simulink model "Proj2"  (R2025a)
settings: Solver=FixedStepDiscrete  StartTime=0.0  StopTime=100.0  FixedStep=0.01  RelTol=1e-3  EnableMultiTasking=on
undefined symbols (not defined in the file): A_total, b, c, DiscIntNeverNeededParam, T_dif, T_get, T_off, T_on, x0
settings Model: SILPILModeSetting=veronly  CodeVerificationMode=processor-in-the-loop (pil)  ExtModeTrigDuration=2  Creator=Lenovo  LastModifiedBy=Sina
settings SolverCC: AutoInsertRateTranBlk=on
settings OptimizationCC: EnhancedBackFolding=on  PassReuseOutputArgsAs=Individual arguments  ZeroExternalMemoryAtStartup=off  ZeroInternalMemoryAtStartup=off  MaxStackSize=64  OptimizeBlockOrder=speed  DifferentSizesBufferReuse=on  OptimizationCustomize=off  EfficientTunableParamExpr=on
settings DebuggingCC: ParameterTunabilityLossMsg=error
settings HardwareCC: ProdBitPerInt=16.0  ProdBitPerPointer=16.0  ProdBitPerSizeT=16.0  ProdBitPerPtrDiffT=16.0  ProdLargestAtomicFloat=None  ProdWordSize=8.0  ProdHWDeviceType=Atmel->AVR
settings SFSimCC: MATLABDynamicMemAlloc=off
settings RTWCC: SystemTargetFile=ert.tlc  HardwareBoard=Arduino Uno  GenCodeOnly=on  TemplateMakefile=ert_default_tmf  Toolchain=Arduino AVR  BuildConfiguration=Faster Runs  Description=Embedded Coder
settings CodeAppCC: ForceParamTrailComments=on  IgnoreCustomStorageClasses=off  OperatorAnnotations=on  SimulinkDataObjDesc=on  SFDataObjDesc=on  InsertBlockDesc=on
settings ERTTargetCC: ExtModeTransport=3.0  ExtModeAutomaticAllocSize=off  ExtModeStaticAllocSize=250.0  InlinedParameterPlacement=Hierarchical  SupportContinuousTime=on  SupportVariableSizeSignals=on
settings ConfigComp: CovEnable=on  RecordCoverage=on  CovModelRefEnable=on

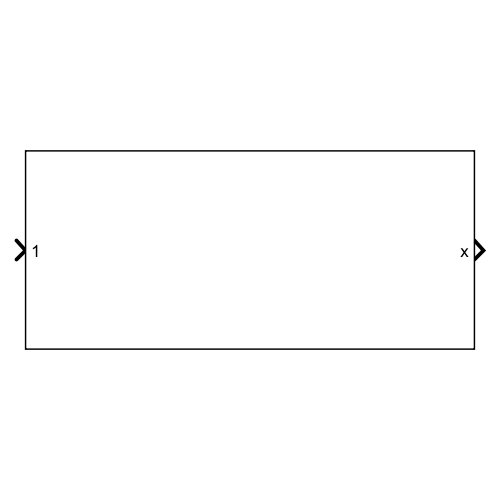
[thumbnail: Simulink's stored preview of the top-level diagram]
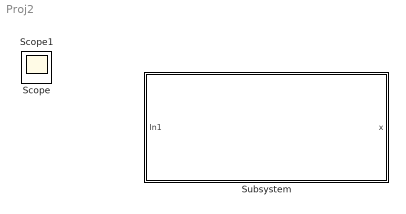
== system Proj2 ==
  Subsystem : Subsystem
  Scope : Scope
      settings: ActiveDisplayYMinimum=12.503923149289818  ActiveDisplayYMaximum=22.756897729507291
  Scope1 : Scope
      settings: ActiveDisplayYMinimum=-4.0864043294794055  ActiveDisplayYMaximum=5.4144619829626475

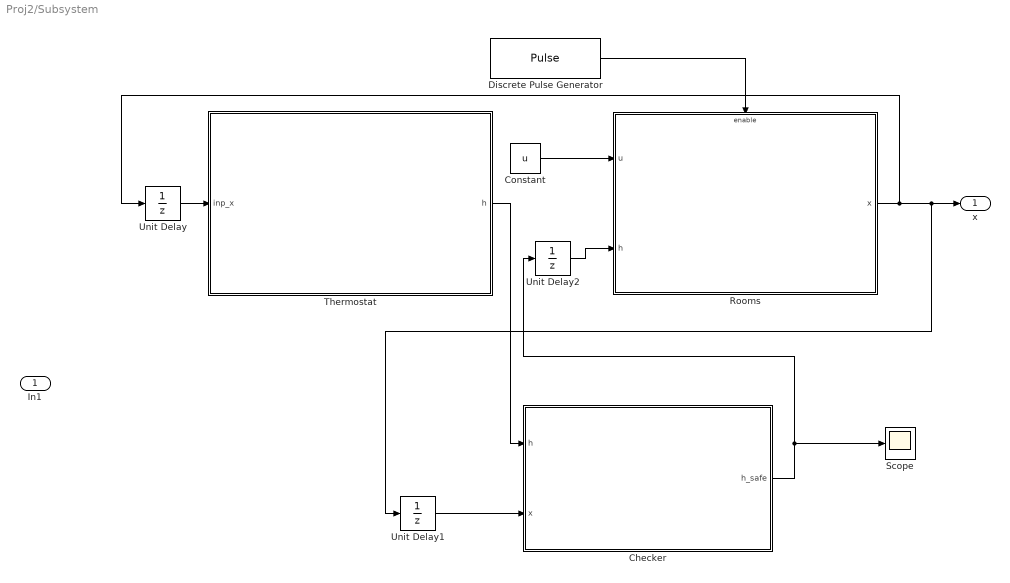
== system Proj2/Subsystem ==
  In1 : Inport
  Checker : Subsystem
  Constant : Constant  Value=u
  Discrete Pulse Generator : DiscretePulseGenerator  PulseType=Time based  Period=1  PulseWidth=50
  Rooms : Subsystem
  Scope : Scope
      settings: ActiveDisplayYMinimum=-0.12499999999999997  ActiveDisplayYMaximum=1.125  DataLoggingVariableName=ScopeData2
  Thermostat : Subsystem
  Unit Delay : UnitDelay  SampleTime=-1  HasFrameUpgradeWarning=on
  Unit Delay1 : UnitDelay  SampleTime=-1  HasFrameUpgradeWarning=on
  Unit Delay2 : UnitDelay  SampleTime=-1  HasFrameUpgradeWarning=on
  x : Outport
  wires:
  Constant/1 -> Rooms/1(u)
  Rooms/1(x) -> Unit Delay/1, Unit Delay1/1, x/1
  Discrete Pulse Generator/1 -> Rooms/Enable
  Unit Delay/1 -> Thermostat/1(inp_x)
  Unit Delay2/1 -> Rooms/2(h)
  Checker/1(h_safe) -> Scope/1, Unit Delay2/1
  Thermostat/1(h) -> Checker/1(h)
  Unit Delay1/1 -> Checker/2(x)

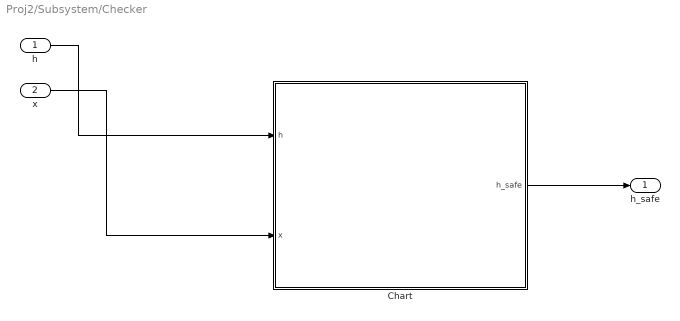
== system Proj2/Subsystem/Checker ==
  h : Inport
  x : Inport  Port=2
  Chart : Stateflow chart  TreatAsAtomicUnit=on
  h_safe : Outport
  wires:
  h/1 -> Chart/1(h)
  Chart/1(h_safe) -> h_safe/1
  x/1 -> Chart/2(x)

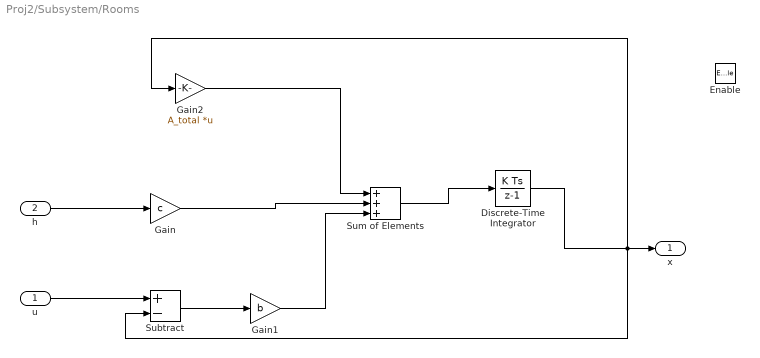
== system Proj2/Subsystem/Rooms ==
  u : Inport
  h : Inport  Port=2
  Enable : EnablePort
  Discrete-Time Integrator : DiscreteIntegrator  InitialCondition=x0  SampleTime=-1  ICPrevOutput=DiscIntNeverNeededParam  ICPrevScaledInput=DiscIntNeverNeededParam
  Gain : Gain  Gain=c
  Gain1 : Gain  Gain=b
  Gain2 : Gain  Gain=A_total  Multiplication=Matrix(K*u)
  Subtract : Sum  Inputs=+-
  Sum of Elements : Sum  Inputs=+++
  x : Outport
  wires:
  Discrete-Time Integrator/1 -> Gain2/1, Subtract/2, x/1
  h/1 -> Gain/1
  u/1 -> Subtract/1
  Subtract/1 -> Gain1/1
  Gain2/1 -> Sum of Elements/1
  Gain/1 -> Sum of Elements/2
  Gain1/1 -> Sum of Elements/3
  Sum of Elements/1 -> Discrete-Time Integrator/1

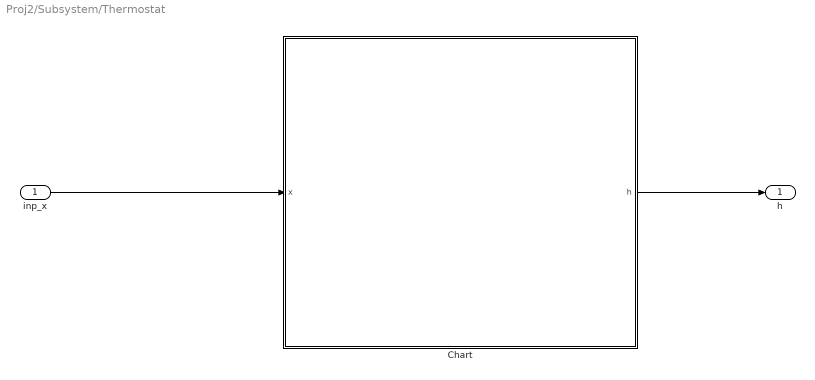
== system Proj2/Subsystem/Thermostat ==
  inp_x : Inport
  Chart : Stateflow chart  TreatAsAtomicUnit=on
  h : Outport
  wires:
  Chart/1(h) -> h/1
  inp_x/1 -> Chart/1(x)

== stateflow chart Proj2/Subsystem/Checker/Chart ==
  state Block
  state Safe
  Block -> Safe [order 1] : [sum(h)<=2]{h_safe = h}
  Safe -> Safe [order 2] : [sum(h)<=2]{h_safe = h}
  (default) -> Block
  Block -> Block [order 2] : [sum(h) > 2 || any((h==1 & x>=T_off) | (h==0 & x<=T_on))]
  Safe -> Block [order 1] : [sum(h) > 2 || any((h==1 & x>=T_off) | (h==0 & x<=T_on))]
  data: h input; h_safe output size=[4 1] =[0;0;0;0]; T_off parameter; T_on parameter; x input

== stateflow chart Proj2/Subsystem/Thermostat/Chart ==
  settings: updateMethod=DISCRETE  sampleTime=0.01
  state S0110
    state S3
    (default) -> S0110.S3
    S0110.S3 -> S0110.S3 [order 4] : [x(2)>=T_off(2) && h(2) == 1]{h(2) = 0;}
    S0110.S3 -> S0110.S3 [order 3] : [x(2) <=T_on(2) && h(2) == 0]{h(2) = 1;}
    S0110.S3 -> S0110.S3 [order 2] : [x(3) <=T_on(3) && h(3) == 0]{h(3) = 1;}
    S0110.S3 -> S0110.S3 [order 1] : [x(3)>=T_off(3) && h(3) == 1]{h(3) = 0;}
  state S1100
    state S3
    (default) -> S1100.S3
    S1100.S3 -> S1100.S3 [order 4] : [x(2)>=T_off(2) && h(2) == 1]{h(2) = 0;}
    S1100.S3 -> S1100.S3 [order 3] : [x(2) <=T_on(2) && h(2) == 0]{h(2) = 1;}
    S1100.S3 -> S1100.S3 [order 2] : [x(1) <=T_on(1) && h(1) == 0]{h(1) = 1;}
    S1100.S3 -> S1100.S3 [order 1] : [x(1)>=T_off(1) && h(1) == 1]{h(1) = 0;}
  state S0011
    state S3
    (default) -> S0011.S3
    S0011.S3 -> S0011.S3 [order 4] : [x(4)>=T_off(4) && h(4) == 1]{h(4) = 0;}
    S0011.S3 -> S0011.S3 [order 3] : [x(4) <=T_on(4) && h(4) == 0]{h(4) = 1;}
    S0011.S3 -> S0011.S3 [order 2] : [x(3) <=T_on(3) && h(3) == 0]{h(3) = 1;}
    S0011.S3 -> S0011.S3 [order 1] : [x(3)>=T_off(3) && h(3) == 1]{h(3) = 0;}
  state S0101
    state S3
    (default) -> S0101.S3
    S0101.S3 -> S0101.S3 [order 4] : [x(2)>=T_off(2) && h(2) == 1]{h(2) = 0;}
    S0101.S3 -> S0101.S3 [order 3] : [x(2) <=T_on(2) && h(2) == 0]{h(2) = 1;}
    S0101.S3 -> S0101.S3 [order 2] : [x(4) <=T_on(4) && h(4) == 0]{h(4) = 1;}
    S0101.S3 -> S0101.S3 [order 1] : [x(4)>=T_off(4) && h(4) == 1]{h(4) = 0;}
  state S1010
    state S3
    (default) -> S1010.S3
    S1010.S3 -> S1010.S3 [order 4] : [x(3)>=T_off(3) && h(3) == 1]{h(3) = 0;}
    S1010.S3 -> S1010.S3 [order 3] : [x(3) <=T_on(3) && h(3) == 0]{h(3) = 1;}
    S1010.S3 -> S1010.S3 [order 2] : [x(1) <=T_on(1) && h(1) == 0]{h(1) = 1;}
    S1010.S3 -> S1010.S3 [order 1] : [x(1)>=T_off(1) && h(1) == 1]{h(1) = 0;}
  state S1001
    state S3
    (default) -> S1001.S3
    S1001.S3 -> S1001.S3 [order 2] : [x(4)>=T_off(4) && h(4) == 1]{h(4) = 0;}
    S1001.S3 -> S1001.S3 [order 1] : [x(4) <=T_on(4) && h(4) == 0]{h(4) = 1;}
    S1001.S3 -> S1001.S3 [order 4] : [x(1) <=T_on(1) && h(1) == 0]{h(1) = 1;}
    S1001.S3 -> S1001.S3 [order 3] : [x(1)>=T_off(1) && h(1) == 1]{h(1) = 0;}
  S0101 -> S0110 [order 1] : [x(3) <=T_get(3) && x(4) - x(3) >= T_dif(3)]{h(4) = 0; h(3) = 1;}
  (default) -> S0110
  S0110 -> S0101 [order 2] : [x(4) <=T_get(4) && x(3) - x(4) >= T_dif(4)]{h(3) = 0; h(4) = 1;}
  S0110 -> S1010 [order 3] : [x(1) <=T_get(1) && x(2) - x(1) >= T_dif(1)]{h(2) = 0; h(1) = 1;}
  S0110 -> S1100 [order 1] : [x(1) <=T_get(1) && x(3) - x(1) >= T_dif(1)]{h(3) = 0; h(1) = 1;}
  S1100 -> S0110 [order 1] : [x(3) <=T_get(3) && x(1) - x(3) >= T_dif(3)]{h(1) = 0; h(3) = 1;}
  S1010 -> S0110 [order 1] : [x(2) <=T_get(2) && x(1) - x(2) >= T_dif(2)]{h(1) = 0; h(2) = 1;}
  S0110 -> S0011 [order 4] : [x(4) <=T_get(4) && x(2) - x(4) >= T_dif(4)]{h(2) = 0; h(4) = 1;}
  S0011 -> S0110 [order 1] : [x(2) <=T_get(2) && x(4) - x(2) >= T_dif(2)]{h(4) = 0; h(2) = 1;}
  S1001 -> S0011 [order 4] : [x(3) <=T_get(3) && x(1) - x(3) >= T_dif(3)]{h(1) = 0; h(3) = 1;}
  S0011 -> S0101 [order 3] : [x(2) <=T_get(2) && x(3) - x(2) >= T_dif(2)]{h(3) = 0; h(2) = 1;}
  S1010 -> S1100 [order 4] : [x(2) <=T_get(2) && x(3) - x(2) >= T_dif(2)]{h(3) = 0; h(2) = 1;}
  S0101 -> S1100 [order 2] : [x(1) <=T_get(1) && x(4) - x(1) >= T_dif(1)]{h(4) = 0; h(1) = 1;}
  S1001 -> S1100 [order 3] : [x(2) <=T_get(2) && x(4) - x(2) >= T_dif(2)]{h(4) = 0; h(2) = 1;}
  S1100 -> S1001 [order 4] : [x(4) <=T_get(4) && x(2) - x(4) >= T_dif(4)]{h(2) = 0; h(4) = 1;}
  S1100 -> S0101 [order 2] : [x(4) <=T_get(4) && x(1) - x(4) >= T_dif(4)]{h(1) = 0; h(4) = 1;}
  S1100 -> S1010 [order 3] : [x(3) <=T_get(3) && x(2) - x(3) >= T_dif(3)]{h(2) = 0; h(3) = 1;}
  S0101 -> S0011 [order 4] : [x(3) <=T_get(3) && x(2) - x(3) >= T_dif(3)]{h(2) = 0; h(3) = 1;}
  S0011 -> S1001 [order 4] : [x(1) <=T_get(1) && x(3) - x(1) >= T_dif(1)]{h(3) = 0; h(1) = 1;}
  S1010 -> S0011 [order 2] : [x(4) <=T_get(4) && x(1) - x(4) >= T_dif(4)]{h(1) = 0; h(4) = 1;}
  S0011 -> S1010 [order 2] : [x(1) <=T_get(1) && x(4) - x(1) >= T_dif(1)]{h(4) = 0; h(1) = 1;}
  S1001 -> S0101 [order 1] : [x(2) <=T_get(2) && x(1) - x(2) >= T_dif(2)]{h(1) = 0; h(2) = 1;}
  S1001 -> S1010 [order 2] : [x(3) <=T_get(3) && x(4) - x(3) >= T_dif(3)]{h(4) = 0; h(3) = 1;}
  S0101 -> S1001 [order 3] : [x(1) <=T_get(1) && x(2) - x(1) >= T_dif(1)]{h(2) = 0; h(1) = 1;}
  S1010 -> S1001 [order 3] : [x(4) <=T_get(4) && x(3) - x(4) >= T_dif(4)]{h(3) = 0; h(4) = 1;}
  data: h output double size=4 =[0; 1; 1; 0]; T_on parameter; T_off parameter; T_get parameter; T_dif parameter; x input
